simulink model "Fuzzy_Manobra"  (R2023b)
settings: Solver=ode45  StartTime=0.0  StopTime=117  FixedStep=0.01  RelTol=1e-9  EnableMultiTasking=on
values from neighbouring files (symbols this model uses):
  b = 0.015    [Inicializar_Qbot2.m]    (also in Inicializar_simulink.m = modelo(7); modelo_PSO_simulink.m = x(7))
  dl = 0    [Inicializar_Qbot2.m]    (also in Inicializar_simulink.m = modelo(3); modelo_PSO_simulink.m = x(3))
  I = Ic+mc*dl^2+2*mw*L^2+2*Im    (= 0.0237413352273)    [Inicializar_Qbot2.m]    (also in Inicializar_simulink.m = modelo(10); modelo_PSO_simulink.m = x(10))
  K = 10.913e-3    (= 0.010913)    [Inicializar_Qbot2.m]    (also in Inicializar_simulink.m = modelo(6); modelo_PSO_simulink.m = x(6))
  L = D/2    (= 0.175)    [Inicializar_Qbot2.m]    (also in Inicializar_simulink.m = modelo(4); modelo_PSO_simulink.m = x(4))
  m = 3.79    [Inicializar_Qbot2.m]    (also in Inicializar_simulink.m = modelo(2); modelo_PSO_simulink.m = x(2))
  R = 0.034    [Inicializar_Qbot2.m]    (also in Inicializar_simulink.m = modelo(1); modelo_PSO_simulink.m = x(1))
  Res = 1.5506    [Inicializar_Qbot2.m]    (also in Inicializar_simulink.m = modelo(8); modelo_PSO_simulink.m = x(8))
undefined symbols (not defined in the file or in its folder): magnitude
libraries: simulink x4, fuzblock x1
settings Model: SimulationMode=rapid-accelerator  ExtModeTrigDuration=100  Creator=Thiago  LastModifiedBy=Gabriel Sousa
settings SolverCC: AlgebraicLoopSolver=TrustRegion
settings DataIOCC: LimitDataPoints=on  SaveFinalState=on  SaveFormat=StructureWithTime  SaveOutput=off  SaveState=on  ReturnWorkspaceOutputs=off  StateSaveName=tmp_raccel_xout  SignalLoggingName=tmp_raccel_logsout
settings OptimizationCC: EfficientMapNaN2IntZero=off  LifeSpan=inf
settings DebuggingCC: UnconnectedInputMsg=warning  UnconnectedOutputMsg=warning  UnconnectedLineMsg=warning  AllowSymbolicDim=off  SFUnexpectedBacktrackingDiag=warning  SFNoUnconditionalDefaultTransitionDiag=warning  SFExecutionAtInitializationDiag=none  ArithmeticOperatorsInVariantConditions=warning
settings HardwareCC: ProdBitPerPointer=32  ProdBitPerSizeT=32  ProdBitPerPtrDiffT=32  ProdLargestAtomicFloat=None  ProdIntDivRoundTo=Undefined  ProdEndianess=Unspecified  ProdWordSize=32  ProdHWDeviceType=32-bit Generic  TargetBitPerPointer=64  TargetBitPerSizeT=64  TargetBitPerPtrDiffT=64  TargetLongLongMode=on  TargetIntDivRoundTo=Zero  TargetEndianess=LittleEndian  TargetWordSize=64  TargetHWDeviceType=MATLAB Host  ProdEqTarget=off
settings ModelReferenceCC: EnableRefExpFcnMdlSchedulingChecks=on  PropagateSignalLabelsOutOfModel=off
settings SFSimCC: SimUseLocalCustomCode=off  CustomCodeUndefinedFunction=UseInterfaceOnly
settings RTWCC: SystemTargetFile=raccel.tlc  TemplateMakefile=raccel_default_tmf  RTWVerbose=off  RTWUseLocalCustomCode=off  RTWUseSimCustomCode=on
settings CodeAppCC: GenerateComments=off  MaxIdLength=128  MangleLength=10
settings RaccelTargetCC: OptimizeReductions=off  ENABLE_SLEXEC_SSBRIDGE=1  RTWCAPIParams=on  RTWCAPIRootIO=off
settings ConfigComp: CovMetricSettings=dw  CovSaveCumulativeToWorkspaceVar=on  CovSaveSingleToWorkspaceVar=on  CovExternalEMLEnable=off
settings SimscapeCC: SimscapeNormalizeSystem=off
settings ConfigurationSet: Description=SimMechanics 2G

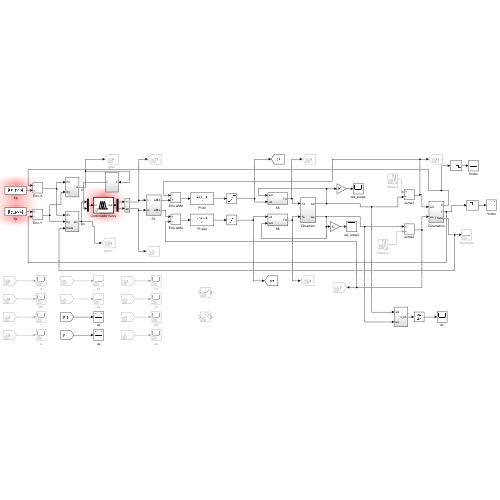
[thumbnail: Simulink's stored preview of the top-level diagram]
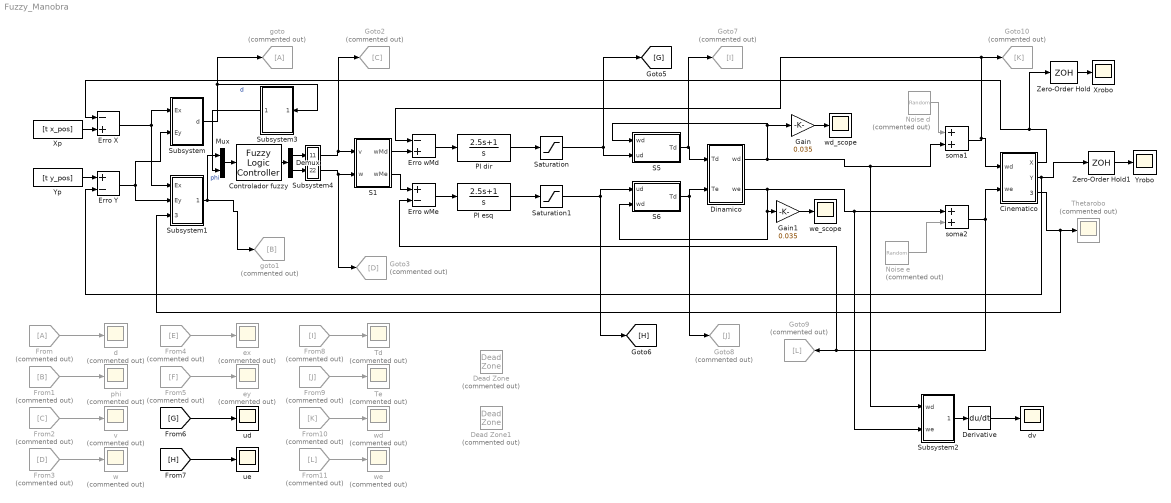
== system Fuzzy_Manobra ==
  Cinematico : Subsystem
  Controlador fuzzy : fuzblock/Fuzzy Logic  Controller  FIS=FB  OutputSampleNumber=101  DataType=double  FuzzifiedInputs=off  RuleFiringStrengths=off  RuleOutputs=off  AggregatedOutputs=off  SimulateUsing=Interpreted execution  OutOfRangeInputValueMessage=warning  NoRuleFiredMessage=warning  EmptyOutputFuzzySetMessage=warning
  Dead Zone : DeadZone  Commented=on  LowerValue=-6  UpperValue=6
  Dead Zone1 : DeadZone  Commented=on  LowerValue=-6  UpperValue=6
  Demux : Demux  Outputs=2
  Derivative : Derivative
  Dinamico : Subsystem
  Erro X : Sum  Inputs=-+
  Erro Y : Sum  Inputs=+-
  Erro wMd : Sum  Inputs=-+
  Erro wMe : Sum  Inputs=+-
  From : From  Commented=on
  From1 : From  Commented=on  GotoTag=B
  From10 : From  Commented=on  GotoTag=K
  From11 : From  Commented=on  GotoTag=L
  From2 : From  Commented=on  GotoTag=C
  From3 : From  Commented=on  GotoTag=D
  From4 : From  Commented=on  GotoTag=E
  From5 : From  Commented=on  GotoTag=F
  From8 : From  Commented=on  GotoTag=I
  From9 : From  Commented=on  GotoTag=J
  Gain : Gain  Gain=0.035
  Gain1 : Gain  Gain=0.035
  Goto10 : Goto  Commented=on  GotoTag=K
  Goto2 : Goto  Commented=on  GotoTag=C
  Goto3 : Goto  Commented=on  GotoTag=D
  Goto7 : Goto  Commented=on  GotoTag=I
  Goto8 : Goto  Commented=on  GotoTag=J
  Goto9 : Goto  Commented=on  GotoTag=L
  Mux : Mux  Inputs=2
  Noise d : RandomNumber  Commented=on  Variance=0.080402  Seed=1  SampleTime=1e-3
  Noise e : RandomNumber  Commented=on  Variance=0.060665  Seed=1  SampleTime=1e-3
  PI dir : TransferFcn  Numerator=[2.5 1]  Denominator=[1 0]
  PI esq : TransferFcn  Numerator=[2.5 1]  Denominator=[1 0]
  S1 : Subsystem
  S5 : Subsystem
  S6 : Subsystem
  Saturation : Saturate  UpperLimit=12  LowerLimit=-12
  Saturation1 : Saturate  UpperLimit=12  LowerLimit=-12
  Subsystem : Subsystem
  Subsystem1 : Subsystem
  Subsystem2 : Subsystem
  Subsystem3 : Subsystem
  Subsystem4 : Subsystem
  Td : Scope  Commented=on
  Te : Scope  Commented=on
  Thetarobo : Scope  Commented=on
  Xp : FromWorkspace  VariableName=[t x_pos]  SampleTime=-1
  Xrobo : Scope
  Yp : FromWorkspace  VariableName=[t y_pos]  SampleTime=-1
  Yrobo : Scope
  Zero-Order Hold : ZeroOrderHold  SampleTime=0.01
  Zero-Order Hold1 : ZeroOrderHold  SampleTime=0.01
  d : Scope  Commented=on
  dv : Scope
  ex : Scope  Commented=on
  ey : Scope  Commented=on
  goto : Goto  Commented=on
  goto1 : Goto  Commented=on  GotoTag=B
  phi : Scope  Commented=on
  soma1 : Sum
  soma2 : Sum
  ud : Scope
  ue : Scope
  v : Scope  Commented=on
  w : Scope  Commented=on
  wd : Scope  Commented=on
  wd_scope : Scope
  we : Scope  Commented=on
  we_scope : Scope
  wires:
  Erro X/1 -> Subsystem1/1(Ex), Subsystem/1(Ex)
  Erro Y/1 -> Subsystem1/2(Ey), Subsystem/2(Ey)
  Erro wMd/1 -> PI dir/1
  Erro wMe/1 -> PI esq/1
  Mux/1 -> Controlador fuzzy/1
  Subsystem1/1(phi) -> Mux/1, goto1/1  "phi"
  Yp/1 -> Erro Y/1
  Xp/1 -> Erro X/2
  Controlador fuzzy/1 -> Demux/1
  S1/1(wMd) -> Erro wMd/2
  S1/2(wMe) -> Erro wMe/1
  Cinematico/3(Theta) -> Thetarobo/1, Subsystem1/3(theta)
  From3/1 -> w/1
  From2/1 -> v/1
  From1/1 -> phi/1
  From/1 -> d/1
  soma2/1 -> Cinematico/2(we), Erro wMe/2, Goto9/1
  soma1/1 -> Cinematico/1(wd), Goto10/1, Erro wMd/1
  Noise e/1 -> soma2/2
  Noise d/1 -> soma1/1
  From5/1 -> ey/1
  From4/1 -> ex/1
  [H] -> ue/1
  [G] -> ud/1
  From8/1 -> Td/1
  From9/1 -> Te/1
  Cinematico/2(Y) -> Erro Y/2, Zero-Order Hold1/1
  PI esq/1 -> Saturation1/1
  PI dir/1 -> Saturation/1
  From10/1 -> wd/1
  From11/1 -> we/1
  Subsystem/1(d) -> Subsystem3/1(In1), goto/1  "d"
  S5/1(Td) -> Dinamico/1(Td), Goto7/1
  S6/1(Td) -> Dinamico/2(Te), Goto8/1
  Subsystem3/1(Out1) -> Mux/2
  Dinamico/2(we) -> Gain1/1, S6/2(wd), Subsystem2/2(we), soma2/1
  Demux/1 -> Subsystem4/1(In1)
  Demux/2 -> Subsystem4/2(In2)
  Subsystem4/1(Out1) -> Goto2/1, S1/1(v)
  Subsystem4/2(Out2) -> Goto3/1, S1/2(w)
  Saturation/1 -> [G], S5/2(ud)
  Saturation1/1 -> S6/1(ud), [H]
  Gain/1 -> wd_scope/1
  Dinamico/1(wd) -> Gain/1, S5/1(wd), Subsystem2/1(wd), soma1/2
  Gain1/1 -> we_scope/1
  Cinematico/1(X) -> Zero-Order Hold/1, Erro X/1
  Zero-Order Hold/1 -> Xrobo/1
  Zero-Order Hold1/1 -> Yrobo/1
  Subsystem2/1(v_lin) -> Derivative/1
  Derivative/1 -> dv/1

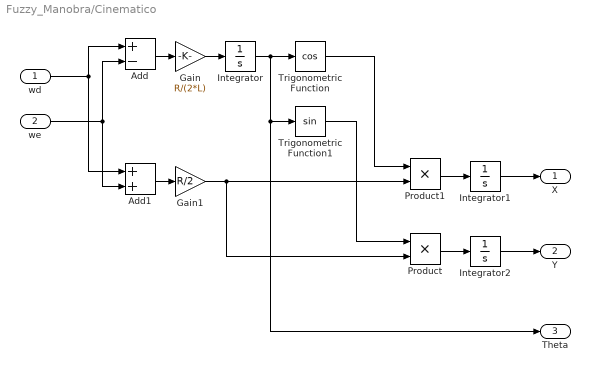
== system Fuzzy_Manobra/Cinematico ==
  wd : Inport
  we : Inport  Port=2
  Add : Sum  Inputs=+-
  Add1 : Sum
  Gain : Gain  Gain=R/(2*L)
  Gain1 : Gain  Gain=R/2
  Integrator : Integrator
  Integrator1 : Integrator
  Integrator2 : Integrator
  Product : Product
  Product1 : Product
  Trigonometric Function : Trigonometry  Operator=cos
  Trigonometric Function1 : Trigonometry
  X : Outport  VectorParamsAs1DForOutWhenUnconnected=off
  Y : Outport  Port=2  VectorParamsAs1DForOutWhenUnconnected=off
  Theta : Outport  Port=3  VectorParamsAs1DForOutWhenUnconnected=off
  wires:
  wd/1 -> Add/1, Add1/1
  we/1 -> Add/2, Add1/2
  Add/1 -> Gain/1
  Gain/1 -> Integrator/1
  Integrator/1 -> Theta/1, Trigonometric Function1/1, Trigonometric Function/1
  Add1/1 -> Gain1/1
  Gain1/1 -> Product/2, Product1/2
  Trigonometric Function/1 -> Product1/1
  Trigonometric Function1/1 -> Product/1
  Product/1 -> Integrator2/1
  Product1/1 -> Integrator1/1
  Integrator1/1 -> X/1
  Integrator2/1 -> Y/1

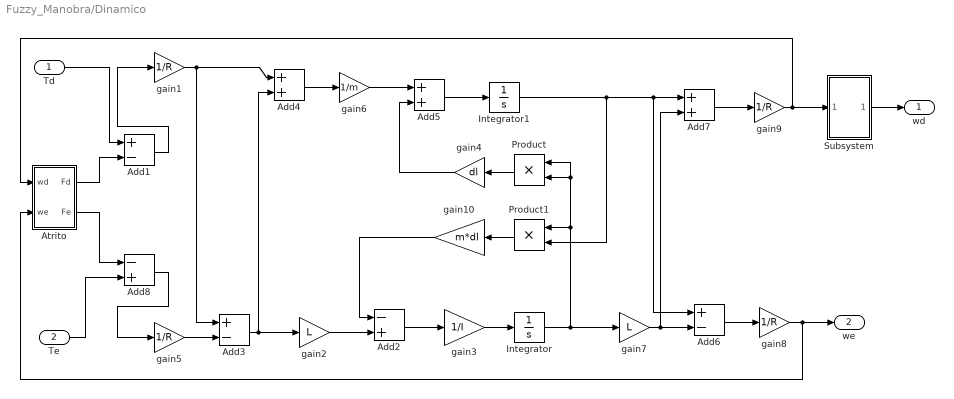
== system Fuzzy_Manobra/Dinamico ==
  Td : Inport
  Te : Inport  Port=2
  Add1 : Sum  Inputs=+-
  Add2 : Sum  Inputs=-+
  Add3 : Sum  Inputs=+-
  Add4 : Sum
  Add5 : Sum
  Add6 : Sum  Inputs=+-
  Add7 : Sum
  Add8 : Sum  Inputs=-+
  Atrito : Subsystem
  Integrator : Integrator
  Integrator1 : Integrator
  Product : Product
  Product1 : Product
  Subsystem : Subsystem
  gain{1,5,8..9} (4 alike) : Gain  Gain=1/R
  gain10 : Gain  Gain=m*dl
  gain2 : Gain  Gain=L
  gain3 : Gain  Gain=1/I
  gain4 : Gain  Gain=dl
  gain6 : Gain  Gain=1/m
  gain7 : Gain  Gain=L
  wd : Outport  VectorParamsAs1DForOutWhenUnconnected=off
  we : Outport  Port=2  VectorParamsAs1DForOutWhenUnconnected=off
  wires:
  gain5/1 -> Add3/2
  gain1/1 -> Add3/1, Add4/1
  Add3/1 -> Add4/2, gain2/1
  Add4/1 -> gain6/1
  gain6/1 -> Add5/1
  gain2/1 -> Add2/2
  Add2/1 -> gain3/1
  gain3/1 -> Integrator/1
  Integrator/1 -> Product1/1, Product/2, Product/1, gain7/1
  gain7/1 -> Add7/2, Add6/2
  Add6/1 -> gain8/1
  Add5/1 -> Integrator1/1
  Integrator1/1 -> Product1/2, Add6/1, Add7/1
  Add7/1 -> gain9/1
  gain4/1 -> Add5/2
  Product/1 -> gain4/1
  Product1/1 -> gain10/1
  gain10/1 -> Add2/1
  Td/1 -> Add1/1
  Te/1 -> Add8/2
  gain8/1 -> Atrito/2(we), we/1
  Add1/1 -> gain1/1
  Atrito/1(Fd) -> Add1/2
  Atrito/2(Fe) -> Add8/1
  Add8/1 -> gain5/1
  gain9/1 -> Subsystem/1(In1), Atrito/1(wd)
  Subsystem/1(Out1) -> wd/1

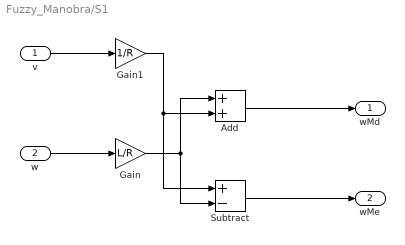
== system Fuzzy_Manobra/S1 ==
  v : Inport
  w : Inport  Port=2
  Add : Sum
  Gain : Gain  Gain=L/R
  Gain1 : Gain  Gain=1/R
  Subtract : Sum  Inputs=+-
  wMd : Outport  VectorParamsAs1DForOutWhenUnconnected=off
  wMe : Outport  Port=2  VectorParamsAs1DForOutWhenUnconnected=off
  wires:
  Subtract/1 -> wMe/1
  Add/1 -> wMd/1
  Gain/1 -> Add/1, Subtract/2
  v/1 -> Gain1/1
  w/1 -> Gain/1
  Gain1/1 -> Add/2, Subtract/1

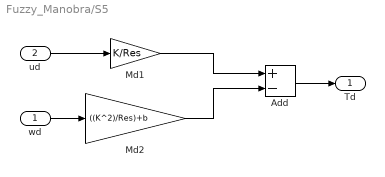
== system Fuzzy_Manobra/S5 ==
  wd : Inport
  ud : Inport  Port=2
  Add : Sum  Inputs=+-
  Md1 : Gain  Gain=K/Res
  Md2 : Gain  Gain=((K^2)/Res)+b
  Td : Outport  VectorParamsAs1DForOutWhenUnconnected=off
  wires:
  Md1/1 -> Add/1
  Md2/1 -> Add/2
  wd/1 -> Md2/1
  ud/1 -> Md1/1
  Add/1 -> Td/1

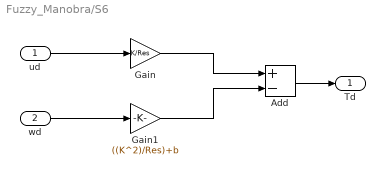
== system Fuzzy_Manobra/S6 ==
  ud : Inport
  wd : Inport  Port=2
  Add : Sum  Inputs=+-
  Gain : Gain  Gain=K/Res
  Gain1 : Gain  Gain=((K^2)/Res)+b
  Td : Outport  VectorParamsAs1DForOutWhenUnconnected=off
  wires:
  Add/1 -> Td/1
  ud/1 -> Gain/1
  wd/1 -> Gain1/1
  Gain1/1 -> Add/2
  Gain/1 -> Add/1

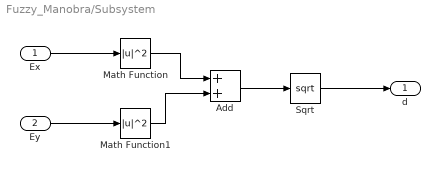
== system Fuzzy_Manobra/Subsystem ==
  Ex : Inport
  Ey : Inport  Port=2
  Add : Sum
  Math Function : Math  Operator=magnitude^2  SignedPower=on
  Math Function1 : Math  Operator=magnitude^2  SignedPower=on
  Sqrt : Sqrt
  d : Outport  VectorParamsAs1DForOutWhenUnconnected=off
  wires:
  Math Function/1 -> Add/1
  Ey/1 -> Math Function1/1
  Add/1 -> Sqrt/1
  Ex/1 -> Math Function/1
  Sqrt/1 -> d/1
  Math Function1/1 -> Add/2

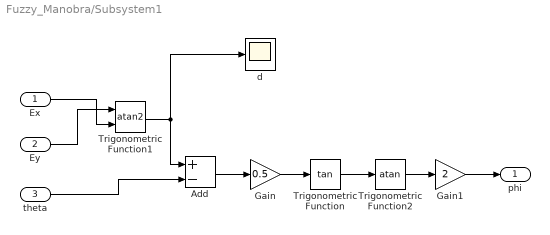
== system Fuzzy_Manobra/Subsystem1 ==
  Ex : Inport
  Ey : Inport  Port=2
  theta : Inport  Port=3
  Add : Sum  Inputs=+-
  Gain : Gain  Gain=0.5
  Gain1 : Gain  Gain=2
  Trigonometric Function : Trigonometry  Operator=tan
  Trigonometric Function1 : Trigonometry  Operator=atan2
  Trigonometric Function2 : Trigonometry  Operator=atan
  d : Scope
  phi : Outport  VectorParamsAs1DForOutWhenUnconnected=off
  wires:
  Ey/1 -> Trigonometric Function1/1
  Ex/1 -> Trigonometric Function1/2
  Trigonometric Function1/1 -> Add/1, d/1
  theta/1 -> Add/2
  Trigonometric Function/1 -> Trigonometric Function2/1
  Trigonometric Function2/1 -> Gain1/1
  Gain/1 -> Trigonometric Function/1
  Gain1/1 -> phi/1
  Add/1 -> Gain/1

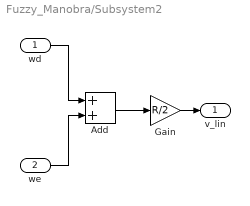
== system Fuzzy_Manobra/Subsystem2 ==
  wd : Inport
  we : Inport  Port=2
  Add : Sum
  Gain : Gain  Gain=R/2
  v_lin : Outport  VectorParamsAs1DForOutWhenUnconnected=off
  wires:
  Add/1 -> Gain/1
  we/1 -> Add/2
  wd/1 -> Add/1
  Gain/1 -> v_lin/1

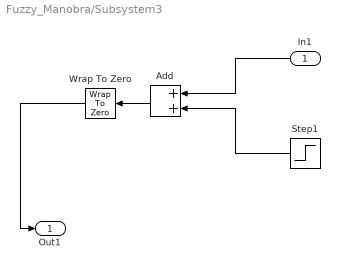
== system Fuzzy_Manobra/Subsystem3 ==
  In1 : Inport
  Add : Sum
  Step1 : Step  Time=t(end-1)  After=50  SampleTime=0
  Wrap To Zero : simulink/Discontinuities/Wrap To Zero  Threshold=50
  Out1 : Outport  VectorParamsAs1DForOutWhenUnconnected=off
  wires:
  Step1/1 -> Add/2
  Add/1 -> Wrap To Zero/1
  In1/1 -> Add/1
  Wrap To Zero/1 -> Out1/1

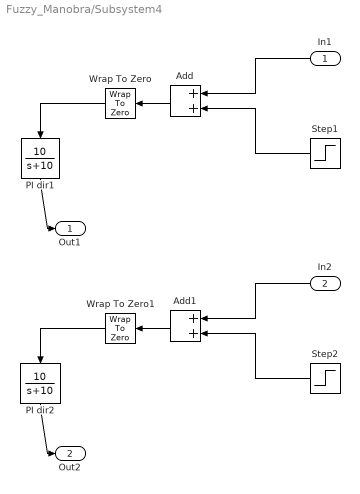
== system Fuzzy_Manobra/Subsystem4 ==
  In1 : Inport
  In2 : Inport  Port=2
  Add : Sum
  Add1 : Sum
  PI dir1 : TransferFcn  Numerator=[10]  Denominator=[1 10]
  PI dir2 : TransferFcn  Numerator=[10]  Denominator=[1 10]
  Step1 : Step  Time=t(end-1)  After=50  SampleTime=0
  Step2 : Step  Time=t(end-1)  After=50  SampleTime=0
  Wrap To Zero : simulink/Discontinuities/Wrap To Zero  Threshold=30
  Wrap To Zero1 : simulink/Discontinuities/Wrap To Zero  Threshold=30
  Out1 : Outport  VectorParamsAs1DForOutWhenUnconnected=off
  Out2 : Outport  Port=2  VectorParamsAs1DForOutWhenUnconnected=off
  wires:
  In1/1 -> Add/1
  Add/1 -> Wrap To Zero/1
  Step1/1 -> Add/2
  Wrap To Zero/1 -> PI dir1/1
  In2/1 -> Add1/1
  Add1/1 -> Wrap To Zero1/1
  Step2/1 -> Add1/2
  Wrap To Zero1/1 -> PI dir2/1
  PI dir1/1 -> Out1/1
  PI dir2/1 -> Out2/1

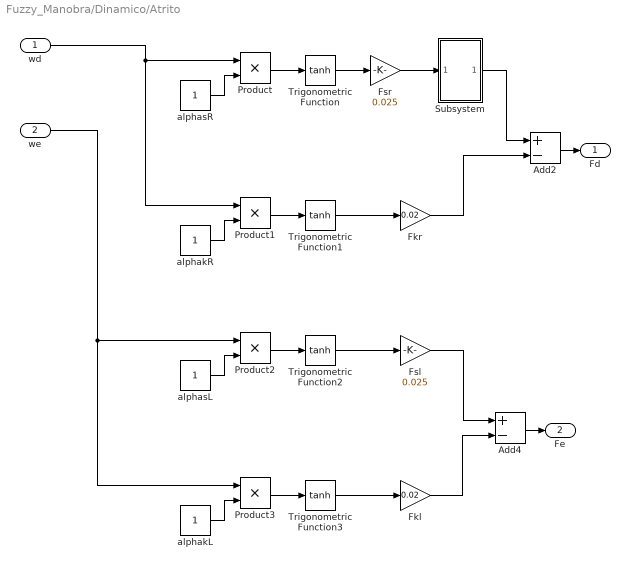
== system Fuzzy_Manobra/Dinamico/Atrito ==
  wd : Inport
  we : Inport  Port=2
  Add2 : Sum  Inputs=+-
  Add4 : Sum  Inputs=+-
  Fkl : Gain  Gain=0.02
  Fkr : Gain  Gain=0.02
  Fsl : Gain  Gain=0.025
  Fsr : Gain  Gain=0.025
  Product{,1..3} (4 alike) : Product
  Subsystem : Subsystem
  Trigonometric Function{,1..3} (4 alike) : Trigonometry  Operator=tanh
  alphakL : Constant
  alphakR : Constant
  alphasL : Constant
  alphasR : Constant
  Fd : Outport  VectorParamsAs1DForOutWhenUnconnected=off
  Fe : Outport  Port=2  VectorParamsAs1DForOutWhenUnconnected=off
  wires:
  we/1 -> Product2/1, Product3/1
  wd/1 -> Product/1, Product1/1
  Fsl/1 -> Add4/1
  Trigonometric Function2/1 -> Fsl/1
  Trigonometric Function/1 -> Fsr/1
  Fkl/1 -> Add4/2
  Trigonometric Function3/1 -> Fkl/1
  Trigonometric Function1/1 -> Fkr/1
  Fkr/1 -> Add2/2
  alphakL/1 -> Product3/2
  Product3/1 -> Trigonometric Function3/1
  Product2/1 -> Trigonometric Function2/1
  alphasL/1 -> Product2/2
  alphasR/1 -> Product/2
  Add4/1 -> Fe/1
  Add2/1 -> Fd/1
  Product1/1 -> Trigonometric Function1/1
  alphakR/1 -> Product1/2
  Product/1 -> Trigonometric Function/1
  Fsr/1 -> Subsystem/1(In1)
  Subsystem/1(Out1) -> Add2/1

== system Fuzzy_Manobra/Dinamico/Subsystem ==
  In1 : Inport
  Add9 : Sum
  Pulse Generator : DiscretePulseGenerator  PulseType=Time based  Amplitude=100  Period=200  PulseWidth=0.8  PhaseDelay=45
  Wrap To Zero : simulink/Discontinuities/Wrap To Zero  Threshold=80
  Out1 : Outport  VectorParamsAs1DForOutWhenUnconnected=off
  wires:
  Add9/1 -> Wrap To Zero/1
  Wrap To Zero/1 -> Out1/1
  In1/1 -> Add9/1

== system Fuzzy_Manobra/Dinamico/Atrito/Subsystem ==
  In1 : Inport
  Add1 : Sum
  Pulse Generator : DiscretePulseGenerator  PulseType=Time based  Amplitude=0.075  Period=200  PulseWidth=2.5  PhaseDelay=220
  Out1 : Outport  VectorParamsAs1DForOutWhenUnconnected=off
  wires:
  Add1/1 -> Out1/1
  In1/1 -> Add1/1
